simulink model "justK"  (R2022b)
settings: Solver=VariableStepAuto  StartTime=0.0  StopTime=10.0  RelTol=1e-3
values from neighbouring files (symbols this model uses):
  K = acker(A,B, [sk sk sk])    [params.m]
settings Model: Creator=antek  LastModifiedBy=antekgrajek

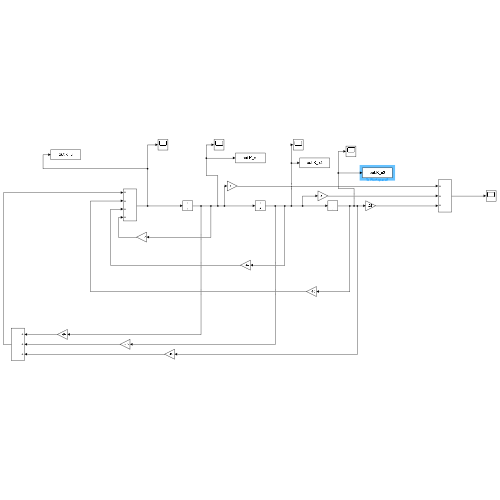
[thumbnail: Simulink's stored preview of the top-level diagram]
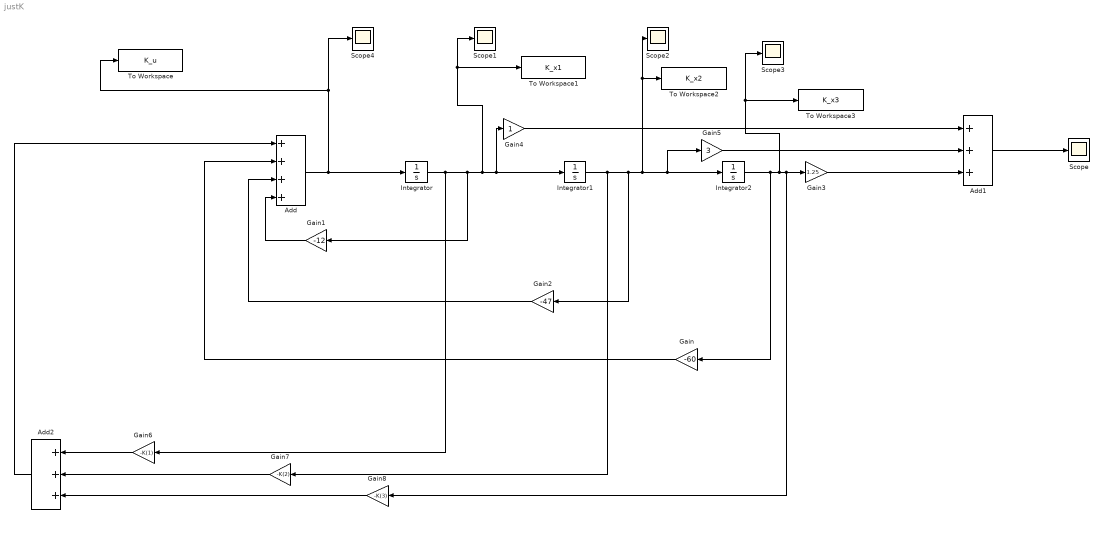
== system justK ==
  Add : Sum  Inputs=++++
  Add1 : Sum  Inputs=+++
  Add2 : Sum  Inputs=+++
  Gain : Gain  Gain=-60
  Gain1 : Gain  Gain=-12
  Gain2 : Gain  Gain=-47
  Gain3 : Gain  Gain=1.25
  Gain4 : Gain
  Gain5 : Gain  Gain=3
  Gain6 : Gain  Gain=-K(1)
  Gain7 : Gain  Gain=-K(2)
  Gain8 : Gain  Gain=-K(3)
  Integrator : Integrator  InitialCondition=5
  Integrator1 : Integrator  InitialCondition=6
  Integrator2 : Integrator  InitialCondition=1
  Scope{,1..4} (5 alike) : Scope
  To Workspace : ToWorkspace  VariableName=K_u  SaveFormat=Timeseries  SampleTime=-1
  To Workspace1 : ToWorkspace  VariableName=K_x1  SaveFormat=Timeseries  SampleTime=-1
  To Workspace2 : ToWorkspace  VariableName=K_x2  SaveFormat=Timeseries  SampleTime=-1
  To Workspace3 : ToWorkspace  VariableName=K_x3  SaveFormat=Timeseries  SampleTime=-1
  wires:
  Gain5/1 -> Add1/2
  Gain/1 -> Add/2
  Gain4/1 -> Add1/1
  Integrator1/1 -> Gain7/1, Gain2/1, To Workspace2/1, Scope2/1, Gain5/1, Integrator2/1
  Gain3/1 -> Add1/3
  Add/1 -> To Workspace/1, Scope4/1, Integrator/1
  Gain2/1 -> Add/3
  Add1/1 -> Scope/1
  Gain1/1 -> Add/4
  Integrator/1 -> Gain6/1, Gain1/1, To Workspace1/1, Scope1/1, Gain4/1, Integrator1/1
  Gain6/1 -> Add2/1
  Gain7/1 -> Add2/2
  Gain8/1 -> Add2/3
  Add2/1 -> Add/1
  Integrator2/1 -> Gain/1, To Workspace3/1, Scope3/1, Gain8/1, Gain3/1
